simulink model "PIDcontroller2023b"  (R2024b)
settings: Solver=VariableStepAuto  StartTime=0.0  StopTime=50  RelTol=1e-3
libraries: spsFirstOrderFilterLib x6, simulink_extras x6
settings Model: Creator=t692s578  LastModifiedBy=tiger
settings RTWCC: GPUComputeCapability=3.5

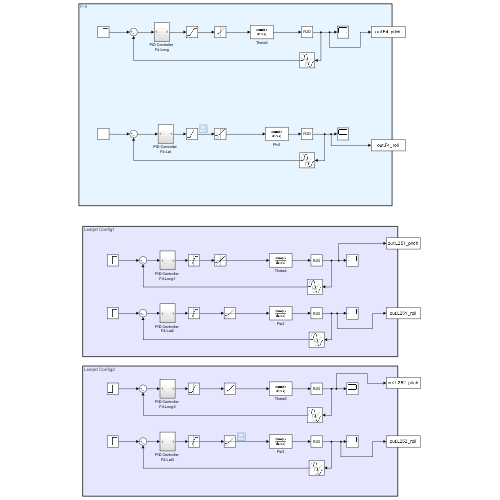
[thumbnail: Simulink's stored preview of the top-level diagram]
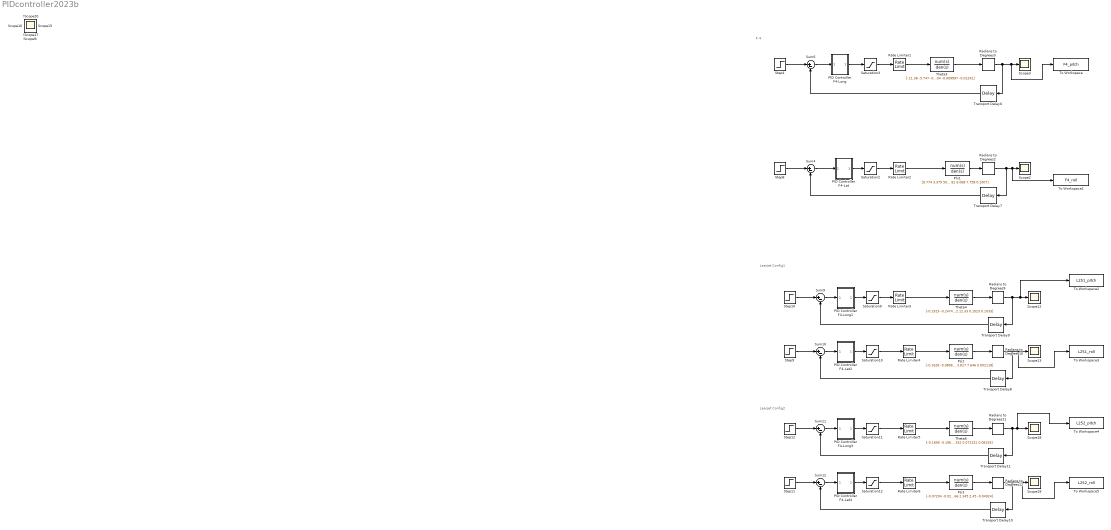
== system PIDcontroller2023b ==
  note: F-4
  note: Learjet Config1
  note: Learjet Config2
  PID Controller F4-Lat : Subsystem
  PID Controller F4-Lat2 : Subsystem
  PID Controller F4-Lat3 : Subsystem
  PID Controller F4-Long : Subsystem
  PID Controller F4-Long1 : Subsystem
  PID Controller F4-Long3 : Subsystem
  Phi1 : TransferFcn  Numerator=[9.774 3.379 50.2]  Denominator=[1 1.581 6.068 7.758 0.1007]
  Psi2 : TransferFcn  Numerator=[-0.1628 -0.08063 -0.4614]  Denominator=[1 2.72 3.817 7.646 0.002118]
  Psi3 : TransferFcn  Numerator=[-0.07204 -0.02628 0.1395]  Denominator=[1 1.366 2.345 2.45 -0.04924]
  Radians to Degrees{2..3,9..12} (6 alike) : simulink_extras/Transformations/Radians to Degrees
  Rate Limiter{1..6} (6 alike) : RateLimiter  RisingSlewLimit=60  FallingSlewLimit=-60  SampleTimeMode=inherited
  Saturation{2..3,9..12} (6 alike) : Saturate  UpperLimit=15  LowerLimit=-15
  Scope{2..3,9..20} (14 alike) : Scope
  Step{4,8..12} (6 alike) : Step  SampleTime=0
  Sum{4,6,9..12} (6 alike) : Sum  Inputs=|+-
  Theta3 : TransferFcn  Numerator=[-11.38 -5.747 -0.06639]  Denominator=[1 1.257 8.104 -0.009997 -0.01242]
  Theta4 : TransferFcn  Numerator=[-0.1919 -0.2474 -0.00406]  Denominator=[1 3.092 12.33 0.1023 0.1033]
  Theta6 : TransferFcn  Numerator=[-0.1856 -0.1962 0.003189]  Denominator=[1 2.706 9.332 0.072151 0.08193]
  To Workspace : ToWorkspace  VariableName=F4_pitch  SaveFormat=Structure With Time  SampleTime=-1
      settings: Save2DSignal=2-D array (concatenate along first dimension)
  To Workspace1 : ToWorkspace  VariableName=F4_roll  SaveFormat=Structure With Time  SampleTime=-1
      settings: Save2DSignal=2-D array (concatenate along first dimension)
  To Workspace2 : ToWorkspace  VariableName=L251_pitch  SaveFormat=Structure With Time  SampleTime=-1
      settings: Save2DSignal=2-D array (concatenate along first dimension)
  To Workspace3 : ToWorkspace  VariableName=L251_roll  SaveFormat=Structure With Time  SampleTime=-1
      settings: Save2DSignal=2-D array (concatenate along first dimension)
  To Workspace4 : ToWorkspace  VariableName=L252_pitch  SaveFormat=Structure With Time  SampleTime=-1
      settings: Save2DSignal=2-D array (concatenate along first dimension)
  To Workspace5 : ToWorkspace  VariableName=L252_roll  SaveFormat=Structure With Time  SampleTime=-1
      settings: Save2DSignal=2-D array (concatenate along first dimension)
  Transport Delay{6..11} (6 alike) : TransportDelay  DelayTime=0.005
  wires:
  Step8/1 -> Sum4/1
  Step4/1 -> Sum6/1
  PID Controller F4-Long/1(Out1) -> Saturation3/1
  Sum6/1 -> PID Controller F4-Long/1(In1)
  Radians to Degrees2/1 -> Transport Delay7/1, To Workspace1/1, Scope2/1
  PID Controller F4-Lat/1(Out1) -> Saturation2/1
  Sum4/1 -> PID Controller F4-Lat/1(In1)
  Radians to Degrees3/1 -> Transport Delay6/1, To Workspace/1, Scope3/1
  Theta3/1 -> Radians to Degrees3/1
  Rate Limiter1/1 -> Theta3/1
  Saturation3/1 -> Rate Limiter1/1
  Saturation2/1 -> Rate Limiter2/1
  Rate Limiter2/1 -> Phi1/1
  Phi1/1 -> Radians to Degrees2/1
  Transport Delay6/1 -> Sum6/2
  Transport Delay7/1 -> Sum4/2
  Step10/1 -> Sum9/1
  Psi2/1 -> Radians to Degrees10/1
  Radians to Degrees10/1 -> To Workspace3/1, Scope13/1, Transport Delay8/1
  Saturation10/1 -> Rate Limiter4/1
  PID Controller F4-Lat2/1(Out1) -> Saturation10/1
  Rate Limiter3/1 -> Theta4/1
  Theta4/1 -> Radians to Degrees9/1
  Step9/1 -> Sum10/1
  Transport Delay8/1 -> Sum10/2
  Radians to Degrees9/1 -> To Workspace2/1, Scope12/1, Transport Delay9/1
  Saturation9/1 -> Rate Limiter3/1
  Sum9/1 -> PID Controller F4-Long1/1(In1)
  PID Controller F4-Long1/1(Out1) -> Saturation9/1
  Sum10/1 -> PID Controller F4-Lat2/1(In1)
  Rate Limiter4/1 -> Psi2/1
  Transport Delay9/1 -> Sum9/2
  Theta6/1 -> Radians to Degrees11/1
  Saturation11/1 -> Rate Limiter5/1
  PID Controller F4-Lat3/1(Out1) -> Saturation12/1
  Sum12/1 -> PID Controller F4-Lat3/1(In1)
  Radians to Degrees12/1 -> To Workspace5/1, Scope19/1, Transport Delay10/1
  Saturation12/1 -> Rate Limiter6/1
  Sum11/1 -> PID Controller F4-Long3/1(In1)
  Rate Limiter5/1 -> Theta6/1
  Psi3/1 -> Radians to Degrees12/1
  Transport Delay10/1 -> Sum12/2
  Radians to Degrees11/1 -> To Workspace4/1, Scope18/1, Transport Delay11/1
  Step11/1 -> Sum12/1
  PID Controller F4-Long3/1(Out1) -> Saturation11/1
  Step12/1 -> Sum11/1
  Rate Limiter6/1 -> Psi3/1
  Transport Delay11/1 -> Sum11/2

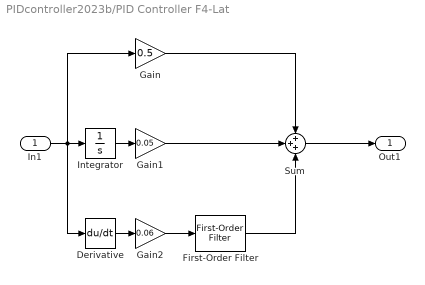
== system PIDcontroller2023b/PID Controller F4-Lat ==
  In1 : Inport
  Derivative : Derivative
  First-Order Filter : spsFirstOrderFilterLib/First-Order Filter  FilterType=Lowpass  Tc=5e-10  Ts=0  Initialize=off  Vac_Init=[0, 0, 60]  Vdc_Init=0  PlotResponse=off  FreqRange="[0,  200,  1]"
  Gain : Gain  Gain=0.5
  Gain1 : Gain  Gain=0.05
  Gain2 : Gain  Gain=0.06
  Integrator : Integrator
  Sum : Sum  Inputs=+++
  Out1 : Outport
  wires:
  In1/1 -> Derivative/1, Gain/1, Integrator/1
  Derivative/1 -> Gain2/1
  Integrator/1 -> Gain1/1
  Gain1/1 -> Sum/2
  Gain/1 -> Sum/1
  Gain2/1 -> First-Order Filter/1
  First-Order Filter/1 -> Sum/3
  Sum/1 -> Out1/1

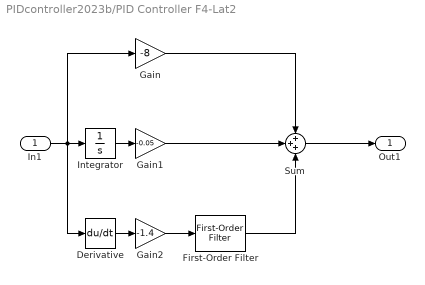
== system PIDcontroller2023b/PID Controller F4-Lat2 ==
  In1 : Inport
  Derivative : Derivative
  First-Order Filter : spsFirstOrderFilterLib/First-Order Filter  FilterType=Lowpass  Tc=5e-3  Ts=0  Initialize=off  Vac_Init=[0, 0, 60]  Vdc_Init=0  PlotResponse=off  FreqRange="[0,  200,  1]"
  Gain : Gain  Gain=-8
  Gain1 : Gain  Gain=-0.05
  Gain2 : Gain  Gain=-1.4
  Integrator : Integrator
  Sum : Sum  Inputs=+++
  Out1 : Outport
  wires:
  In1/1 -> Derivative/1, Gain/1, Integrator/1
  Derivative/1 -> Gain2/1
  Integrator/1 -> Gain1/1
  Gain1/1 -> Sum/2
  Gain/1 -> Sum/1
  Gain2/1 -> First-Order Filter/1
  First-Order Filter/1 -> Sum/3
  Sum/1 -> Out1/1

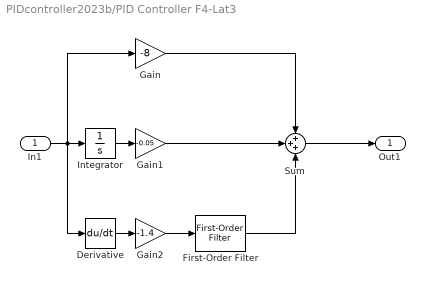
== system PIDcontroller2023b/PID Controller F4-Lat3 ==
  In1 : Inport
  Derivative : Derivative
  First-Order Filter : spsFirstOrderFilterLib/First-Order Filter  FilterType=Lowpass  Tc=5e-3  Ts=0  Initialize=off  Vac_Init=[0, 0, 60]  Vdc_Init=0  PlotResponse=off  FreqRange="[0,  200,  1]"
  Gain : Gain  Gain=-8
  Gain1 : Gain  Gain=-0.05
  Gain2 : Gain  Gain=-1.4
  Integrator : Integrator
  Sum : Sum  Inputs=+++
  Out1 : Outport
  wires:
  In1/1 -> Derivative/1, Gain/1, Integrator/1
  Derivative/1 -> Gain2/1
  Integrator/1 -> Gain1/1
  Gain1/1 -> Sum/2
  Gain/1 -> Sum/1
  Gain2/1 -> First-Order Filter/1
  First-Order Filter/1 -> Sum/3
  Sum/1 -> Out1/1

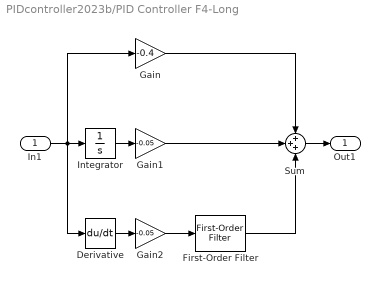
== system PIDcontroller2023b/PID Controller F4-Long ==
  In1 : Inport
  Derivative : Derivative
  First-Order Filter : spsFirstOrderFilterLib/First-Order Filter  FilterType=Lowpass  Tc=5e-6  Ts=0  Initialize=off  Vac_Init=[0, 0, 60]  Vdc_Init=0  PlotResponse=off  FreqRange="[0,  200,  1]"
  Gain : Gain  Gain=-0.4
  Gain1 : Gain  Gain=-0.05
  Gain2 : Gain  Gain=-0.05
  Integrator : Integrator
  Sum : Sum  Inputs=+++
  Out1 : Outport
  wires:
  In1/1 -> Derivative/1, Gain/1, Integrator/1
  Derivative/1 -> Gain2/1
  Integrator/1 -> Gain1/1
  Gain2/1 -> First-Order Filter/1
  First-Order Filter/1 -> Sum/3
  Gain1/1 -> Sum/2
  Gain/1 -> Sum/1
  Sum/1 -> Out1/1

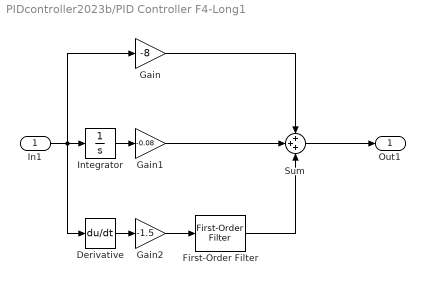
== system PIDcontroller2023b/PID Controller F4-Long1 ==
  In1 : Inport
  Derivative : Derivative
  First-Order Filter : spsFirstOrderFilterLib/First-Order Filter  FilterType=Lowpass  Tc=5e-5  Ts=0  Initialize=off  Vac_Init=[0, 0, 60]  Vdc_Init=0  PlotResponse=off  FreqRange="[0,  200,  1]"
  Gain : Gain  Gain=-8
  Gain1 : Gain  Gain=-0.08
  Gain2 : Gain  Gain=-1.5
  Integrator : Integrator
  Sum : Sum  Inputs=+++
  Out1 : Outport
  wires:
  In1/1 -> Derivative/1, Gain/1, Integrator/1
  Derivative/1 -> Gain2/1
  Integrator/1 -> Gain1/1
  Gain1/1 -> Sum/2
  Gain/1 -> Sum/1
  Gain2/1 -> First-Order Filter/1
  First-Order Filter/1 -> Sum/3
  Sum/1 -> Out1/1

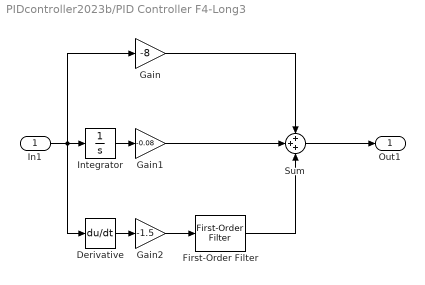
== system PIDcontroller2023b/PID Controller F4-Long3 ==
  In1 : Inport
  Derivative : Derivative
  First-Order Filter : spsFirstOrderFilterLib/First-Order Filter  FilterType=Lowpass  Tc=5e-5  Ts=0  Initialize=off  Vac_Init=[0, 0, 60]  Vdc_Init=0  PlotResponse=off  FreqRange="[0,  200,  1]"
  Gain : Gain  Gain=-8
  Gain1 : Gain  Gain=-0.08
  Gain2 : Gain  Gain=-1.5
  Integrator : Integrator
  Sum : Sum  Inputs=+++
  Out1 : Outport
  wires:
  In1/1 -> Derivative/1, Gain/1, Integrator/1
  Derivative/1 -> Gain2/1
  Integrator/1 -> Gain1/1
  Gain1/1 -> Sum/2
  Gain/1 -> Sum/1
  Gain2/1 -> First-Order Filter/1
  First-Order Filter/1 -> Sum/3
  Sum/1 -> Out1/1
